simulink model "eVTOL_System"  (R2024b)
settings: Solver=FixedStepAuto  StartTime=0.0  StopTime=inf  RelTol=1e-3
undefined symbols (not defined in the file): airspeed, Battery, BCE12, BCE_Set_init, BMS_Controller_State, C, Cell10_P, Cell11_P, Cell12_P, Cell13_P, Cell14_P, Cell15_P, Cell16_P, Cell17_P, Cell18_P, Cell19_P, Cell1_N, Cell1_P, Cell20_P, Cell21_P, Cell22_P, Cell23_P, Cell24_P, Cell2_P, Cell3_P, Cell4_P, Cell5_P, Cell6_P, Cell7_P, Cell8_P, Cell9_P, Charging_State, CityMission, control, controlParams, ControlSampleTime, CriticalTiltAngle, currentFactor, CV_Gain, ddx, ddy, ddz, Device_01, Device_02, DiscIntNeverNeededParam, dx, dy, dz, Earth, env, F, F28379D_ADC_MaxCount, F28379D_ADC_Vmax, FixedWingMission, flightState, Foc_Ki_IxTcpu, Foc_Ki_S, Foc_Kp_I, Foc_Kp_S, fractalcoef ... (+68)
libraries: fl_lib x1115, nesl_utility x617, slrealtimeethercatlib x217, simulink x130, canmsglib x101, speedgoatlib_IO611_obsolete x91, slpidlib x49, mcbcontrolslib x44, slrealtimeutilitieslib x35, speedgoatlib_hdlCoder_IO3xx x31, dspstat3 x24, mcbpositiondecoderlib x12
(part 11 of 31)

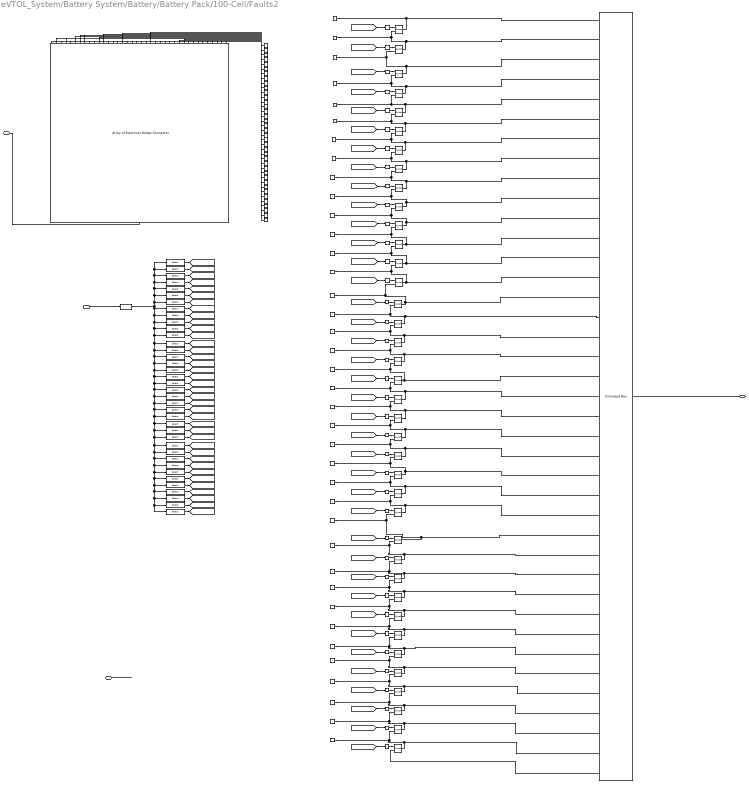
== system eVTOL_System/Battery System/Battery/Battery Pack/100-Cell/Faults2 ==
  note: Short-Circuits
  note: Short-Circuits
  note: Short-Circuits
  Short_Circuits : Inport
  Array of Electrical Nodes Connector2 : batt_lib/Connectors/Array of Electrical Nodes Connector  numInputConnections=simscape.battery.enum.thermal.numArrayOfNodesConnections.thirtyeight  inNode1NumElements=1  inNode2NumElements=1  inNode3NumElements=1  inNode4NumElements=1  inNode5NumElements=1  inNode6NumElements=1  inNode7NumElements=1  inNode8NumElements=1  inNode9NumElements=1  inNode10NumElements=1  inNode11NumElements=1  inNode12NumElements=1  inNode13NumElements=1  inNode14NumElements=1  inNode15NumElements=1  inNode16NumElements=1  inNode17NumElements=1  inNode18NumElements=1  inNode19NumElements=1  inNode20NumElements=1  inNode21NumElements=1  inNode22NumElements=1  inNode23NumElements=1  inNode24NumElements=1  inNode25NumElements=1  inNode26NumElements=1  inNode27NumElements=1  inNode28NumElements=1  inNode29NumElements=1  inNode30NumElements=1  inNode31NumElements=1  inNode32NumElements=1  inNode33NumElements=1  inNode34NumElements=1  inNode35NumElements=1  inNode36NumElements=1  inNode37NumElements=1  inNode38NumElements=1  inNode39NumElements=1  inNode40NumElements=1  inNode41NumElements=1  inNode42NumElements=1  inNode43NumElements=1  inNode44NumElements=1  inNode45NumElements=1  inNode46NumElements=1  inNode47NumElements=1  inNode48NumElements=1  inNode49NumElements=1  inNode50NumElements=1
      settings: InternalSimscapePortConfiguration="{\"Bottom\":[{\"id\":\"outConn\",\"label\":\"outConn\",\"type\":\"foundation.electrical.electrical\"}],\"Left\":[],\"Right\":[],\"Top\":[{\"id\":\"inConn1\",\"label\":\"inConn1\",\"type\":\"foundation.electrical.electrical\"},{\"id\":\"inConn2\",\"label\":\"inConn2\",\"type\":\"foundation.electrical.electrical\"},{\"id\":\"inConn3\",\"label\":\"inConn3\",\"type\":\"foundation.electrical.electrical\"},{\"id\":\"inConn4\",\"label\":\"inConn4\",\"type\":\"foundation.electrical.electrical\"},{\"id\":\"inConn5\",\"label\":\"inConn5\",\"type\":\"foundation.electrical.electrical\"},{\"id\":\"inConn6\",\"label\":\"inConn6\",\"type\":\"foundation.electrical.electrical\"},{\"id\":\"inConn7\",\"label\":\"inConn7\",\"type\":\"foundation.electrical.electrical\"},{\"id\":\"inConn8\",\"label\":\"inConn8\",\"type\":\"foundation.electrical.electrical\"},{\"id\":\"inConn9\",\"label\":\"inConn9\",\"type\":\"foundation.electrical.electrical\"},{\"id\":\"inConn10\",\"label\":\"inConn10\",\"type\":\"foundation.electrical.electrical\"},{\"id\":\"inConn11\",\"label\":\"inConn11\",\"type\":\"foundation.electrical.electrical\"},{\"id\":\"inConn12\",\"label\":\"inConn12\",\"type\":\"foundation.electrical.electrical\"},{\"id\":\"inConn13\",\"label\":\"inConn13\",\"type\":\"foundation.electrical.electrical\"},{\"id\":\"inConn14\",\"label\":\"inConn14\",\"type\":\"foundation.electrical.electrical\"},{\"id\":\"inConn15\",\"label\":\"inConn15\",\"type\":\"foundation.electrical.electrical\"},{\"id\":\"inConn16\",\"label\":\"inConn16\",\"type\":\"foundation.electrical.electrical\"},{\"id\":\"inConn17\",\"label\":\"inConn17\",\"type\":\"foundation.electrical.electrical\"},{\"id\":\"inConn18\",\"label\":\"inConn18\",\"type\":\"foundation.electrical.electrical\"},{\"id\":\"inConn19\",\"label\":\"inConn19\",\"type\":\"foundation.electrical.electrical\"},{\"id\":\"inConn20\",\"label\":\"inConn20\",\"type\":\"foundation.electrical.electrical\"},{\"id\":\"inConn21\",\"label\":\"inConn21\",\"type\":\"foundation.electrical.electrical\"},{\"id\":\"inConn22\",\"label\":\"inConn22\",\"type\":\"foundation.electrical.electrical\"},{\"id\":\"inConn23\",\"label\":\"inConn23\",\"type\":\"foundation.electrical.electrical\"},{\"id\":\"inConn24\",\"label\":\"inConn24\",\"type\":\"foundation.electrical.electrical\"},{\"id\":\"inConn25\",\"label\":\"inConn25\",\"type\":\"foundation.electrical.electrical\"},{\"id\":\"inConn26\",\"label\":\"inConn26\",\"type\":\"foundation.electrical.electrical\"},{\"id\":\"inConn27\",\"label\":\"inConn27\",\"type\":\"foundation.electrical.electrical\"},{\"id\":\"inConn28\",\"label\":\"inConn28\",\"type\":\"foundation.electrical.electrical\"},{\"id\":\"inConn29\",\"label\":\"inConn29\",\"type\":\"foundation.electrical.electrical\"},{\"id\":\"inConn30\",\"label\":\"inConn30\",\"type\":\"foundation.electrical.electrical\"},{\"id\":\"inConn31\",\"label\":\"inConn31\",\"type\":\"foundation.electrical.electrical\"},{\"id\":\"inConn32\",\"label\":\"inConn32\",\"type\":\"foundation.electrical.electrical\"},{\"id\":\"inConn33\",\"label\":\"inConn33\",\"type\":\"foundation.electrical.electrical\"},{\"id\":\"inConn34\",\"label\":\"inConn34\",\"type\":\"foundation.electrical.electrical\"},{\"id\":\"inConn35\",\"label\":\"inConn35\",\"type\":\"foundation.electrical.electrical\"},{\"id\":\"inConn36\",\"label\":\"inConn36\",\"type\":\"foundation.electrical.electrical\"},{\"id\":\"inConn37\",\"label\":\"inConn37\",\"type\":\"foundation.electrical.electrical\"},{\"id\":\"inConn38\",\"label\":\"inConn38\",\"type\":\"foundation.electrical.electrical\"}]}"
  Connection Label1 : ConnectionLabel  Label=pos12
  Connection Label10 : ConnectionLabel  Label=pos3
  Connection Label100 : ConnectionLabel  Label=pos1
  Connection Label101 : ConnectionLabel  Label=pos7
  Connection Label102 : ConnectionLabel  Label=pos3
  Connection Label103 : ConnectionLabel  Label=pos2
  Connection Label104 : ConnectionLabel  Label=pos8
  Connection Label105 : ConnectionLabel  Label=pos9
  Connection Label106 : ConnectionLabel  Label=pos10
  Connection Label107 : ConnectionLabel  Label=pos11
  Connection Label108 : ConnectionLabel  Label=pos12
  Connection Label109 : ConnectionLabel  Label=pos6
  Connection Label11 : ConnectionLabel  Label=pos2
  Connection Label110 : ConnectionLabel  Label=pos13
  Connection Label111 : ConnectionLabel  Label=pos19
  Connection Label112 : ConnectionLabel  Label=pos15
  Connection Label113 : ConnectionLabel  Label=pos14
  Connection Label114 : ConnectionLabel  Label=pos20
  Connection Label115 : ConnectionLabel  Label=pos21
  Connection Label116 : ConnectionLabel  Label=pos5
  Connection Label117 : ConnectionLabel  Label=pos22
  Connection Label118 : ConnectionLabel  Label=pos23
  Connection Label119 : ConnectionLabel  Label=pos24
  Connection Label12 : ConnectionLabel  Label=pos1
  Connection Label120 : ConnectionLabel  Label=pos18
  Connection Label121 : ConnectionLabel  Label=pos17
  Connection Label122 : ConnectionLabel  Label=pos16
  Connection Label123 : ConnectionLabel  Label=pos25
  Connection Label124 : ConnectionLabel  Label=pos31
  Connection Label125 : ConnectionLabel  Label=pos27
  Connection Label126 : ConnectionLabel  Label=pos26
  Connection Label127 : ConnectionLabel  Label=pos4
  Connection Label128 : ConnectionLabel  Label=pos32
  Connection Label129 : ConnectionLabel  Label=pos33
  Connection Label13 : ConnectionLabel  Label=pos24
  Connection Label130 : ConnectionLabel  Label=pos34
  Connection Label131 : ConnectionLabel  Label=pos35
  Connection Label132 : ConnectionLabel  Label=pos36
  Connection Label133 : ConnectionLabel  Label=pos30
  Connection Label134 : ConnectionLabel  Label=pos29
  Connection Label135 : ConnectionLabel  Label=pos28
  Connection Label136 : ConnectionLabel  Label=pos37
  Connection Label137 : ConnectionLabel  Label=pos38
  Connection Label14 : ConnectionLabel  Label=pos23
  Connection Label15 : ConnectionLabel  Label=pos22
  Connection Label16 : ConnectionLabel  Label=pos21
  Connection Label17 : ConnectionLabel  Label=pos20
  Connection Label18 : ConnectionLabel  Label=pos19
  Connection Label19 : ConnectionLabel  Label=pos18
  Connection Label2 : ConnectionLabel  Label=pos11
  Connection Label20 : ConnectionLabel  Label=pos17
  Connection Label21 : ConnectionLabel  Label=pos29
  Connection Label22 : ConnectionLabel  Label=pos16
  Connection Label23 : ConnectionLabel  Label=pos15
  Connection Label3 : ConnectionLabel  Label=pos10
  Connection Label4 : ConnectionLabel  Label=pos9
  Connection Label48 : ConnectionLabel  Label=pos14
  Connection Label49 : ConnectionLabel  Label=pos13
  Connection Label5 : ConnectionLabel  Label=pos8
  Connection Label50 : ConnectionLabel  Label=pos28
  Connection Label51 : ConnectionLabel  Label=pos27
  Connection Label52 : ConnectionLabel  Label=pos26
  Connection Label53 : ConnectionLabel  Label=pos25
  Connection Label54 : ConnectionLabel  Label=pos34
  Connection Label55 : ConnectionLabel  Label=pos33
  Connection Label56 : ConnectionLabel  Label=pos32
  Connection Label57 : ConnectionLabel  Label=pos31
  Connection Label58 : ConnectionLabel  Label=pos30
  Connection Label59 : ConnectionLabel  Label=pos38
  Connection Label6 : ConnectionLabel  Label=pos7
  Connection Label60 : ConnectionLabel  Label=pos37
  Connection Label61 : ConnectionLabel  Label=pos36
  Connection Label62 : ConnectionLabel  Label=pos35
  Connection Label7 : ConnectionLabel  Label=pos6
  Connection Label8 : ConnectionLabel  Label=pos5
  Connection Label9 : ConnectionLabel  Label=pos4
  Data Type Conversion2 : DataTypeConversion  OutDataTypeStr=double  SaturateOnIntegerOverflow=off  RndMeth=Floor
  Selector1 : Selector  IndexOptions=Index vector (dialog)  Indices=73  OutputSizes=1
  Selector10 : Selector  IndexOptions=Index vector (dialog)  Indices=63  OutputSizes=1
  Selector11 : Selector  IndexOptions=Index vector (dialog)  Indices=64  OutputSizes=1
  Selector12 : Selector  IndexOptions=Index vector (dialog)  Indices=66  OutputSizes=1
  Selector13 : Selector  IndexOptions=Index vector (dialog)  Indices=76  OutputSizes=1
  Selector14 : Selector  IndexOptions=Index vector (dialog)  Indices=86  OutputSizes=1
  Selector15 : Selector  IndexOptions=Index vector (dialog)  Indices=85  OutputSizes=1
  Selector16 : Selector  IndexOptions=Index vector (dialog)  Indices=83  OutputSizes=1
  Selector17 : Selector  IndexOptions=Index vector (dialog)  Indices=78  OutputSizes=1
  Selector18 : Selector  IndexOptions=Index vector (dialog)  Indices=77  OutputSizes=1
  Selector19 : Selector  IndexOptions=Index vector (dialog)  Indices=80  OutputSizes=1
  Selector2 : Selector  IndexOptions=Index vector (dialog)  Indices=71  OutputSizes=1
  Selector20 : Selector  IndexOptions=Index vector (dialog)  Indices=82  OutputSizes=1
  Selector21 : Selector  IndexOptions=Index vector (dialog)  Indices=75  OutputSizes=1
  Selector22 : Selector  IndexOptions=Index vector (dialog)  Indices=81  OutputSizes=1
  Selector23 : Selector  IndexOptions=Index vector (dialog)  Indices=79  OutputSizes=1
  Selector24 : Selector  IndexOptions=Index vector (dialog)  Indices=84  OutputSizes=1
  Selector25 : Selector  IndexOptions=Index vector (dialog)  Indices=89  OutputSizes=1
  Selector26 : Selector  IndexOptions=Index vector (dialog)  Indices=88  OutputSizes=1
  Selector27 : Selector  IndexOptions=Index vector (dialog)  Indices=91  OutputSizes=1
  Selector29 : Selector  IndexOptions=Index vector (dialog)  Indices=100  OutputSizes=1
  Selector3 : Selector  IndexOptions=Index vector (dialog)  Indices=72  OutputSizes=1
  Selector30 : Selector  IndexOptions=Index vector (dialog)  Indices=98  OutputSizes=1
  Selector31 : Selector  IndexOptions=Index vector (dialog)  Indices=93  OutputSizes=1
  Selector32 : Selector  IndexOptions=Index vector (dialog)  Indices=92  OutputSizes=1
  Selector33 : Selector  IndexOptions=Index vector (dialog)  Indices=95  OutputSizes=1
  Selector34 : Selector  IndexOptions=Index vector (dialog)  Indices=97  OutputSizes=1
  Selector35 : Selector  IndexOptions=Index vector (dialog)  Indices=90  OutputSizes=1
  Selector36 : Selector  IndexOptions=Index vector (dialog)  Indices=96  OutputSizes=1
  Selector37 : Selector  IndexOptions=Index vector (dialog)  Indices=94  OutputSizes=1
  Selector38 : Selector  IndexOptions=Index vector (dialog)  Indices=99  OutputSizes=1
  Selector39 : Selector  IndexOptions=Index vector (dialog)  Indices=87  OutputSizes=1
  Selector4 : Selector  IndexOptions=Index vector (dialog)  Indices=69  OutputSizes=1
  Selector5 : Selector  IndexOptions=Index vector (dialog)  Indices=67  OutputSizes=1
  Selector6 : Selector  IndexOptions=Index vector (dialog)  Indices=74  OutputSizes=1
  Selector7 : Selector  IndexOptions=Index vector (dialog)  Indices=68  OutputSizes=1
  Selector8 : Selector  IndexOptions=Index vector (dialog)  Indices=70  OutputSizes=1
  Selector9 : Selector  IndexOptions=Index vector (dialog)  Indices=65  OutputSizes=1
  Simscape Bus : SimscapeBus  HierarchyStrings=Cell38_P;Cell37_P;Cell36_P;Cell35_P;Cell34_P;Cell33_P;Cell32_P;Cell31_P;Cell30_P;Cell29_P;Cell28_P;Cell27_P;Cell26_P;Cell25_P;Cell24_P;Cell23_P;Cell22_P;Cell21_P;Cell20_P;Cell19_P;Cell18_P;Cell17_P;Cell16_P;Cell15_P;Cell14_P;Cell13_P;Cell12_P;Cell11_P;Cell10_P;Cell9_P;Cell8_P;Cell7_P;Cell6_P;Cell5_P;Cell4_P;Cell3_P;Cell2_P;Cell1_P;Cell1_N
  Simulink-PS Converter{1..38} (38 alike) : nesl_utility/Simulink-PS Converter  PhysicalDomain=network_engine_domain  SubClassName=ps_input  LeftPortType=input  RightPortType=output  PseudoPeriodic=off  Frequencies=[]  NoiseDistribution=none  NoiseParameters=[]  Unit=1  AffineConversion=off  FilteringAndDerivatives=zero  SimscapeFilterOrder=1  InputFilterTimeConstant=0.001  UdotUserProvided=1
  Switch{,1..37} (38 alike) : fl_lib/Electrical/Electrical Elements/Switch  R_closed=0.01 Ohm  G_open=1e-8 1/Ohm  Threshold=0.5  i_specify=off  i_priority=None  i=0 A  i_nominal_specify=off  i_nominal_value=1  i_nominal_unit=A  v_specify=off  v_priority=None  v=0 V  v_nominal_specify=off  v_nominal_value=1  v_nominal_unit=V
  +Bus : PMIOPort  Side=Right
  Cells : PMIOPort  Port=2  Side=Right
  =Bus : PMIOPort  Port=3  Side=Right
  wires:
  [Cell37_Switch_SC] -> Simulink-PS Converter24/1
  [Cell36_Switch_SC] -> Simulink-PS Converter23/1
  [Cell38_Switch_SC] -> Simulink-PS Converter25/1
  [Cell27_Switch_SC] -> Simulink-PS Converter14/1
  [Cell28_Switch_SC] -> Simulink-PS Converter15/1
  [Cell35_Switch_SC] -> Simulink-PS Converter22/1
  [Cell31_Switch_SC] -> Simulink-PS Converter18/1
  [Cell34_Switch_SC] -> Simulink-PS Converter21/1
  [Cell29_Switch_SC] -> Simulink-PS Converter16/1
  [Cell30_Switch_SC] -> Simulink-PS Converter17/1
  [Cell33_Switch_SC] -> Simulink-PS Converter20/1
  [Cell32_Switch_SC] -> Simulink-PS Converter19/1
  [Cell23_Switch_SC] -> Simulink-PS Converter9/1
  [Cell20_Switch_SC] -> Simulink-PS Converter6/1
  [Cell17_Switch_SC] -> Simulink-PS Converter3/1
  [Cell18_Switch_SC] -> Simulink-PS Converter4/1
  [Cell26_Switch_SC] -> Simulink-PS Converter12/1
  [Cell19_Switch_SC] -> Simulink-PS Converter5/1
  [Cell25_Switch_SC] -> Simulink-PS Converter11/1
  [Cell22_Switch_SC] -> Simulink-PS Converter8/1
  [Cell15_Switch_SC] -> Simulink-PS Converter1/1
  [Cell24_Switch_SC] -> Simulink-PS Converter10/1
  [Cell21_Switch_SC] -> Simulink-PS Converter7/1
  [Cell16_Switch_SC] -> Simulink-PS Converter2/1
  [Cell5_Switch_SC] -> Simulink-PS Converter30/1
  [Cell4_Switch_SC] -> Simulink-PS Converter29/1
  [Cell10_Switch_SC] -> Simulink-PS Converter35/1
  [Cell12_Switch_SC] -> Simulink-PS Converter26/1
  [Cell3_Switch_SC] -> Simulink-PS Converter13/1
  [Cell9_Switch_SC] -> Simulink-PS Converter34/1
  [Cell14_Switch_SC] -> Simulink-PS Converter28/1
  [Cell13_Switch_SC] -> Simulink-PS Converter27/1
  [Cell6_Switch_SC] -> Simulink-PS Converter31/1
  [Cell11_Switch_SC] -> Simulink-PS Converter36/1
  [Cell7_Switch_SC] -> Simulink-PS Converter32/1
  [Cell8_Switch_SC] -> Simulink-PS Converter33/1
  [Cell1_Switch_SC] -> Simulink-PS Converter37/1
  Short_Circuits/1 -> Data Type Conversion2/1
  Selector11/1 -> [Cell2_Switch_SC]
  Selector16/1 -> [Cell21_Switch_SC]
  Selector9/1 -> [Cell3_Switch_SC]
  Selector14/1 -> [Cell24_Switch_SC]
  Selector27/1 -> [Cell29_Switch_SC]
  Selector10/1 -> [Cell1_Switch_SC]
  Selector7/1 -> [Cell6_Switch_SC]
  Selector2/1 -> [Cell9_Switch_SC]
  Selector21/1 -> [Cell13_Switch_SC]
  Selector13/1 -> [Cell14_Switch_SC]
  Selector34/1 -> [Cell35_Switch_SC]
  Selector22/1 -> [Cell19_Switch_SC]
  Selector26/1 -> [Cell26_Switch_SC]
  Selector31/1 -> [Cell31_Switch_SC]
  Data Type Conversion2/1 -> Selector5/1, Selector12/1, Selector9/1, Selector11/1, Selector30/1, Selector29/1, Selector38/1, Selector34/1, Selector36/1, Selector33/1, Selector37/1, Selector31/1, Selector32/1, Selector27/1, Selector35/1, Selector25/1, Selector26/1, Selector39/1, Selector14/1, Selector15/1, Selector24/1, Selector16/1, Selector20/1, Selector22/1, Selector19/1, Selector23/1, Selector17/1, Selector18/1, Selector13/1, Selector21/1, Selector10/1, Selector4/1, Selector8/1, Selector2/1, Selector3/1, Selector1/1, Selector6/1, Selector7/1
  Selector35/1 -> [Cell28_Switch_SC]
  Selector25/1 -> [Cell27_Switch_SC]
  Selector36/1 -> [Cell34_Switch_SC]
  Selector18/1 -> [Cell15_Switch_SC]
  Selector33/1 -> [Cell33_Switch_SC]
  Selector39/1 -> [Cell25_Switch_SC]
  Selector17/1 -> [Cell16_Switch_SC]
  Selector37/1 -> [Cell32_Switch_SC]
  Selector32/1 -> [Cell30_Switch_SC]
  Selector24/1 -> [Cell22_Switch_SC]
  Selector30/1 -> [Cell36_Switch_SC]
  Selector38/1 -> [Cell37_Switch_SC]
  Selector23/1 -> [Cell17_Switch_SC]
  Selector20/1 -> [Cell20_Switch_SC]
  Selector19/1 -> [Cell18_Switch_SC]
  Selector29/1 -> [Cell38_Switch_SC]
  Selector15/1 -> [Cell23_Switch_SC]
  Selector6/1 -> [Cell12_Switch_SC]
  Selector5/1 -> [Cell5_Switch_SC]
  Selector12/1 -> [Cell4_Switch_SC]
  Selector8/1 -> [Cell8_Switch_SC]
  Selector4/1 -> [Cell7_Switch_SC]
  Selector1/1 -> [Cell11_Switch_SC]
  Selector3/1 -> [Cell10_Switch_SC]
  [Cell2_Switch_SC] -> Simulink-PS Converter38/1
  connections:
  Simulink-PS Converter17/RConn1 -- Switch3/RConn1
  Switch3/LConn1 -- Simscape Bus/LConn30 -- Switch2/RConn2 -- Connection Label58/LConn1
  Switch6/LConn1 -- Simscape Bus/LConn33 -- Switch5/RConn2 -- Connection Label55/LConn1
  Switch7/LConn1 -- Simscape Bus/LConn34 -- Connection Label54/LConn1 -- Switch6/RConn2
  Switch2/LConn1 -- Simscape Bus/LConn29 -- Switch1/RConn2 -- Connection Label21/LConn1
  Simulink-PS Converter16/RConn1 -- Switch2/RConn1
  Simulink-PS Converter19/RConn1 -- Switch5/RConn1
  Switch10/LConn1 -- Simscape Bus/LConn37 -- Switch9/RConn2 -- Connection Label60/LConn1
  Simulink-PS Converter25/RConn1 -- Switch11/RConn1
  Switch11/LConn1 -- Simscape Bus/LConn38 -- Connection Label59/LConn1 -- Switch10/RConn2
  Switch9/LConn1 -- Simscape Bus/LConn36 -- Switch8/RConn2 -- Connection Label61/LConn1
  Simulink-PS Converter14/RConn1 -- Switch/RConn1
  Simscape Bus/LConn39 -- Switch11/RConn2
  Simulink-PS Converter18/RConn1 -- Switch4/RConn1
  Switch4/LConn1 -- Simscape Bus/LConn31 -- Switch3/RConn2 -- Connection Label57/LConn1
  Simulink-PS Converter24/RConn1 -- Switch10/RConn1
  Switch8/LConn1 -- Simscape Bus/LConn35 -- Switch7/RConn2 -- Connection Label62/LConn1
  Simulink-PS Converter20/RConn1 -- Switch6/RConn1
  Simulink-PS Converter15/RConn1 -- Switch1/RConn1
  Simulink-PS Converter21/RConn1 -- Switch7/RConn1
  Simulink-PS Converter23/RConn1 -- Switch9/RConn1
  Simulink-PS Converter22/RConn1 -- Switch8/RConn1
  Switch5/LConn1 -- Simscape Bus/LConn32 -- Switch4/RConn2 -- Connection Label56/LConn1
  Simscape Bus/LConn27 -- Connection Label51/LConn1 -- Switch15/RConn2 -- Switch/LConn1
  Switch1/LConn1 -- Simscape Bus/LConn28 -- Connection Label50/LConn1 -- Switch/RConn2
  =Bus/RConn1 -- ?
  Switch17/LConn1 -- Simscape Bus/LConn18 -- Switch16/RConn2 -- Connection Label19/LConn1
  Switch14/LConn1 -- Simscape Bus/LConn25 -- Switch23/RConn2 -- Connection Label53/LConn1
  Switch19/LConn1 -- Connection Label17/LConn1 -- Switch18/RConn2 -- Simscape Bus/LConn20
  Switch13/LConn1 -- Simscape Bus/LConn16 -- Switch12/RConn2 -- Connection Label22/LConn1
  Switch22/LConn1 -- Simscape Bus/LConn23 -- Connection Label14/LConn1 -- Switch21/RConn2
  Switch18/LConn1 -- Simscape Bus/LConn19 -- Connection Label18/LConn1 -- Switch17/RConn2
  Switch16/LConn1 -- Simscape Bus/LConn17 -- Connection Label20/LConn1 -- Switch13/RConn2
  Switch12/LConn1 -- Switch27/RConn2 -- Connection Label23/LConn1 -- Simscape Bus/LConn15
  Switch21/LConn1 -- Switch20/RConn2 -- Connection Label15/LConn1 -- Simscape Bus/LConn22
  Simscape Bus/LConn21 -- Switch19/RConn2 -- Connection Label16/LConn1 -- Switch20/LConn1
  Simulink-PS Converter12/RConn1 -- Switch15/RConn1
  Simulink-PS Converter7/RConn1 -- Switch20/RConn1
  Simulink-PS Converter10/RConn1 -- Switch23/RConn1
  Simulink-PS Converter2/RConn1 -- Switch13/RConn1
  Simulink-PS Converter3/RConn1 -- Switch16/RConn1
  Simulink-PS Converter1/RConn1 -- Switch12/RConn1
  Simulink-PS Converter11/RConn1 -- Switch14/RConn1
  Simulink-PS Converter8/RConn1 -- Switch21/RConn1
  Simulink-PS Converter9/RConn1 -- Switch22/RConn1
  Simulink-PS Converter5/RConn1 -- Switch18/RConn1
  Simulink-PS Converter6/RConn1 -- Switch19/RConn1
  Simulink-PS Converter4/RConn1 -- Switch17/RConn1
  Switch15/LConn1 -- Simscape Bus/LConn26 -- Connection Label52/LConn1 -- Switch14/RConn2
  Simscape Bus/LConn24 -- Switch23/LConn1 -- Connection Label13/LConn1 -- Switch22/RConn2
  Cells/RConn1 -- Simscape Bus/RConn1
  Switch33/LConn1 -- Connection Label3/LConn1 -- Switch32/RConn2 -- Simscape Bus/LConn10
  Simscape Bus/LConn3 -- Connection Label10/LConn1 -- Switch37/RConn2 -- Switch24/LConn1
  Switch34/LConn1 -- Simscape Bus/LConn11 -- Connection Label2/LConn1 -- Switch33/RConn2
  Switch25/LConn1 -- Connection Label9/LConn1 -- Switch24/RConn2 -- Simscape Bus/LConn4
  Switch31/LConn1 -- Switch30/RConn2 -- Connection Label5/LConn1 -- Simscape Bus/LConn8
  Simscape Bus/LConn14 -- Switch27/LConn1 -- Switch26/RConn2 -- Connection Label48/LConn1
  Switch26/LConn1 -- Connection Label49/LConn1 -- Switch35/RConn2 -- Simscape Bus/LConn13
  Switch30/LConn1 -- Switch29/RConn2 -- Connection Label6/LConn1 -- Simscape Bus/LConn7
  Switch32/LConn1 -- Switch31/RConn2 -- Connection Label4/LConn1 -- Simscape Bus/LConn9
  Switch29/LConn1 -- Connection Label7/LConn1 -- Switch28/RConn2 -- Simscape Bus/LConn6
  Switch28/LConn1 -- Switch25/RConn2 -- Connection Label8/LConn1 -- Simscape Bus/LConn5
  Switch35/LConn1 -- Connection Label1/LConn1 -- Switch34/RConn2 -- Simscape Bus/LConn12
  Simulink-PS Converter31/RConn1 -- Switch29/RConn1
  Simulink-PS Converter13/RConn1 -- Switch24/RConn1
  Simulink-PS Converter28/RConn1 -- Switch27/RConn1
  Simulink-PS Converter35/RConn1 -- Switch33/RConn1
  Simulink-PS Converter34/RConn1 -- Switch32/RConn1
  Simulink-PS Converter33/RConn1 -- Switch31/RConn1
  Simulink-PS Converter27/RConn1 -- Switch26/RConn1
  Simulink-PS Converter32/RConn1 -- Switch30/RConn1
  Simulink-PS Converter29/RConn1 -- Switch25/RConn1
  Simulink-PS Converter36/RConn1 -- Switch34/RConn1
  Simulink-PS Converter30/RConn1 -- Switch28/RConn1
  Simulink-PS Converter26/RConn1 -- Switch35/RConn1
  Simscape Bus/LConn1 -- Connection Label12/LConn1 -- Switch36/LConn1
  Switch37/LConn1 -- Connection Label11/LConn1 -- Switch36/RConn2 -- Simscape Bus/LConn2
  Simulink-PS Converter37/RConn1 -- Switch36/RConn1
  Simulink-PS Converter38/RConn1 -- Switch37/RConn1
  Connection Label132/LConn1 -- Array of Electrical Nodes Connector2/LConn36
  Connection Label107/LConn1 -- Array of Electrical Nodes Connector2/LConn11
  Connection Label106/LConn1 -- Array of Electrical Nodes Connector2/LConn10
  Connection Label136/LConn1 -- Array of Electrical Nodes Connector2/LConn37
  Connection Label131/LConn1 -- Array of Electrical Nodes Connector2/LConn35
  Connection Label135/LConn1 -- Array of Electrical Nodes Connector2/LConn28
  Connection Label129/LConn1 -- Array of Electrical Nodes Connector2/LConn33
  Connection Label128/LConn1 -- Array of Electrical Nodes Connector2/LConn32
  Connection Label124/LConn1 -- Array of Electrical Nodes Connector2/LConn31
  Connection Label125/LConn1 -- Array of Electrical Nodes Connector2/LConn27
  Connection Label118/LConn1 -- Array of Electrical Nodes Connector2/LConn23
  Connection Label121/LConn1 -- Array of Electrical Nodes Connector2/LConn17
  Connection Label114/LConn1 -- Array of Electrical Nodes Connector2/LConn20
  Connection Label102/LConn1 -- Array of Electrical Nodes Connector2/LConn3
  Connection Label133/LConn1 -- Array of Electrical Nodes Connector2/LConn30
  Connection Label120/LConn1 -- Array of Electrical Nodes Connector2/LConn18
  Connection Label123/LConn1 -- Array of Electrical Nodes Connector2/LConn25
  Connection Label115/LConn1 -- Array of Electrical Nodes Connector2/LConn21
  Connection Label111/LConn1 -- Array of Electrical Nodes Connector2/LConn19
  Connection Label112/LConn1 -- Array of Electrical Nodes Connector2/LConn15
  Connection Label126/LConn1 -- Array of Electrical Nodes Connector2/LConn26
  Connection Label104/LConn1 -- Array of Electrical Nodes Connector2/LConn8
  Connection Label109/LConn1 -- Array of Electrical Nodes Connector2/LConn6
  Connection Label119/LConn1 -- Array of Electrical Nodes Connector2/LConn24
  Connection Label105/LConn1 -- Array of Electrical Nodes Connector2/LConn9
  Connection Label116/LConn1 -- Array of Electrical Nodes Connector2/LConn5
  Connection Label137/LConn1 -- Array of Electrical Nodes Connector2/LConn38
  Connection Label100/LConn1 -- Array of Electrical Nodes Connector2/LConn1
  Connection Label134/LConn1 -- Array of Electrical Nodes Connector2/LConn29
  Connection Label122/LConn1 -- Array of Electrical Nodes Connector2/LConn16
  Connection Label103/LConn1 -- Array of Electrical Nodes Connector2/LConn2
  Connection Label117/LConn1 -- Array of Electrical Nodes Connector2/LConn22
  Connection Label101/LConn1 -- Array of Electrical Nodes Connector2/LConn7
  Connection Label127/LConn1 -- Array of Electrical Nodes Connector2/LConn4
  Connection Label130/LConn1 -- Array of Electrical Nodes Connector2/LConn34
  +Bus/RConn1 -- Array of Electrical Nodes Connector2/RConn1
  Connection Label113/LConn1 -- Array of Electrical Nodes Connector2/LConn14
  Connection Label110/LConn1 -- Array of Electrical Nodes Connector2/LConn13
  Connection Label108/LConn1 -- Array of Electrical Nodes Connector2/LConn12

== system eVTOL_System/Battery System/Battery/Battery Pack/100-Cell/Trigger_Faults ==
  Cell_Number : Constant  Value=12
  Delay : Delay  DelayLength=1
  Enable : Constant  Value=0
  Reset : Constant  Value=0
  Short-Circuit_Faults : MATLAB Function  TreatAsAtomicUnit=on
  ShortCircuit : Outport
  wires:
  Short-Circuit_Faults/1(ShortCircuit) -> Delay/1, ShortCircuit/1
  Cell_Number/1 -> Short-Circuit_Faults/1(CellNumber)
  Enable/1 -> Short-Circuit_Faults/2(Enable)
  Reset/1 -> Short-Circuit_Faults/3(Reset)
  Delay/1 -> Short-Circuit_Faults/4(Feedback)

== system eVTOL_System/Battery System/Battery/HW Interface/BCE - HIL/Battery Cell Emulator ==
  Sensor_Values_Sim : Inport
  "BCE Bus Packing " : Subsystem
  BCE Bus Packing 1 : Subsystem
  "BCE Read " : Subsystem  InitFcn=sg_bce.checkNumberOfBlocksGlobal(bdroot);  mask(bce_read){}
      settings: OpenFcn=sg_bce.openFcnRead;
      mask Help: eval('sg.utils.help.show(''io_main/refentry_bce_read'');')
      mask Display: disp('Speedgoat\nBMTS Read\nEtherCAT Bus: 0, Device: 1\nBCE12-0505');port_label('output',1,'Data');
  BCE Read 1 : Subsystem  InitFcn=sg_bce.checkNumberOfBlocksGlobal(bdroot);  mask(bce_read){}
      settings: OpenFcn=sg_bce.openFcnRead;
      mask Help: eval('sg.utils.help.show(''io_main/refentry_bce_read'');')
      mask Display: disp('Speedgoat\nBMTS Read\nEtherCAT Bus: 0, Device: 2\nBCE12-0505');port_label('output',1,'Data');
  "BCE Setup " : Subsystem  LoadFcn=|  InitFcn=|  mask(bce_setup){}
      LoadFcn=|
      | sg_bce.createBusSignals;
      | sg_bce.setupEniCallback(gcb, bdroot);
      InitFcn=|
      | sg_bce.createBusSignals;
      | sg_bce.checkNumberOfBlocksGlobal(bdroot);
      | sg_bce.setupEniCallback(gcb, bdroot);
      settings: OpenFcn=sg_bce.openFcnSetup;
      mask Help: eval('sg.utils.help.show(''io_main/refentry_bce_setup'');')
      mask Display: disp('Speedgoat\nBattery Management Testing Systems\nEtherCAT Bus: 0\nSetup');
  "BCE Write " : Subsystem  InitFcn=sg_bce.checkNumberOfBlocksGlobal(bdroot);  mask(bce_write){}
      settings: OpenFcn=sg_bce.openFcnWrite;
      mask Help: eval('sg.utils.help.show(''io_main/refentry_bce_write'');')
      mask Display: disp('Speedgoat\nBMTS Write\nEtherCAT Bus: 0, Device: 1\nBCE12-0505');port_label('input',1,'Data');
  BCE Write 1 : Subsystem  InitFcn=sg_bce.checkNumberOfBlocksGlobal(bdroot);  mask(bce_write){}
      settings: OpenFcn=sg_bce.openFcnWrite;
      mask Help: eval('sg.utils.help.show(''io_main/refentry_bce_write'');')
      mask Display: disp('Speedgoat\nBMTS Write\nEtherCAT Bus: 0, Device: 2\nBCE12-0505');port_label('input',1,'Data');
  BCE_Init : Switch  Criteria=u2 > Threshold  SaturateOnIntegerOverflow=off  InputSameDT=off
  Bus Selector : BusSelector  OutputSignals=Cell_12.I,Cell_11.I,Cell_10.I,Cell_9.I,Cell_8.I,Cell_7.I,Cell_6.I,Cell_5.I,Cell_4.I,Cell_3.I,Cell_2.I,Cell_1.I
  Bus Selector2 : BusSelector  OutputSignals=Cell_12.V,Cell_11.V,Cell_10.V,Cell_9.V,Cell_8.V,Cell_7.V,Cell_6.V,Cell_5.V,Cell_4.V,Cell_3.V,Cell_2.V,Cell_1.V
  Bus Selector3 : BusSelector  OutputSignals=Cell_12.I,Cell_11.I,Cell_10.I,Cell_9.I,Cell_8.I,Cell_7.I,Cell_6.I,Cell_5.I,Cell_4.I,Cell_3.I,Cell_2.I,Cell_1.I
  Bus Selector4 : BusSelector  OutputSignals=Cell_12.V,Cell_11.V,Cell_10.V,Cell_9.V,Cell_8.V,Cell_7.V,Cell_6.V,Cell_5.V,Cell_4.V,Cell_3.V,Cell_2.V,Cell_1.V
  Constant : Constant  Value=[0 0 0 0 0 0 0 0 0 0 0 0 0 0 0 0 0 0 0 0 0 0 0 0]
  Data Type Conversion : DataTypeConversion  OutDataTypeStr=single  SaturateOnIntegerOverflow=off  RndMeth=Floor
  Data Type Conversion1 : DataTypeConversion  OutDataTypeStr=boolean  SaturateOnIntegerOverflow=off  RndMeth=Floor
  Data Type Conversion2 : DataTypeConversion  OutDataTypeStr=single  SaturateOnIntegerOverflow=off  RndMeth=Floor
  Data Type Conversion3 : DataTypeConversion  OutDataTypeStr=single  SaturateOnIntegerOverflow=off  RndMeth=Floor
  Data Type Conversion4 : DataTypeConversion  OutDataTypeStr=boolean  SaturateOnIntegerOverflow=off  RndMeth=Floor
  Demux : Demux  Outputs=12
  Demux1 : Demux  Outputs=12
  Enable : Constant
  Enable1 : Constant
  Mux{,1..3} (4 alike) : Mux  Inputs=12
  Mux4 : Mux  Inputs=2
  Mux5 : Mux  Inputs=2
  No_current : Constant  Value=0
  No_current1 : Constant  Value=0
  Selector : Subsystem
  Selector1 : Subsystem
  Selector2 : Subsystem
  Selector3 : Subsystem
  Step : Step  Time=2
  Current_Values : Outport
  Cell_Voltages : Outport  Port=2
  OtherVoltages : Outport  Port=3
  wires:
  "BCE Read "/1(Data) -> Bus Selector/1, Bus Selector2/1
  Constant/1 -> Data Type Conversion2/1
  Step/1 -> BCE_Init/2
  "BCE Bus Packing "/1(BCE Bus) -> "BCE Write "/1(Data)
  No_current/1 -> Data Type Conversion/1
  Data Type Conversion2/1 -> BCE_Init/3
  Bus Selector/1 -> Mux/1  "<I>"
  Bus Selector/2 -> Mux/2  "<I>"
  Bus Selector/3 -> Mux/3  "<I>"
  Bus Selector/4 -> Mux/4  "<I>"
  Bus Selector/5 -> Mux/5  "<I>"
  Bus Selector/6 -> Mux/6  "<I>"
  Bus Selector/7 -> Mux/7  "<I>"
  Bus Selector/8 -> Mux/8  "<I>"
  Bus Selector/9 -> Mux/9  "<I>"
  Bus Selector/10 -> Mux/10  "<I>"
  Bus Selector/11 -> Mux/11  "<I>"
  Bus Selector/12 -> Mux/12  "<I>"
  Bus Selector2/1 -> Mux1/1  "<V>"
  Bus Selector2/2 -> Mux1/2  "<V>"
  Bus Selector2/3 -> Mux1/3  "<V>"
  Bus Selector2/4 -> Mux1/4  "<V>"
  Bus Selector2/5 -> Mux1/5  "<V>"
  Bus Selector2/6 -> Mux1/6  "<V>"
  Bus Selector2/7 -> Mux1/7  "<V>"
  Bus Selector2/8 -> Mux1/8  "<V>"
  Bus Selector2/9 -> Mux1/9  "<V>"
  Bus Selector2/10 -> Mux1/10  "<V>"
  Bus Selector2/11 -> Mux1/11  "<V>"
  Bus Selector2/12 -> Mux1/12  "<V>"
  Enable/1 -> Data Type Conversion1/1
  Data Type Conversion1/1 -> "BCE Bus Packing "/1(Cell 1 Enable), "BCE Bus Packing "/9(Cell 9 Enable), "BCE Bus Packing "/12(Cell 12 Enable), "BCE Bus Packing "/11(Cell 11 Enable), "BCE Bus Packing "/10(Cell 10 Enable), "BCE Bus Packing "/8(Cell 8 Enable), "BCE Bus Packing "/7(Cell 7 Enable), "BCE Bus Packing "/6(Cell 6 Enable), "BCE Bus Packing "/5(Cell 5 Enable), "BCE Bus Packing "/4(Cell 4 Enable), "BCE Bus Packing "/3(Cell 3 Enable), "BCE Bus Packing "/2(Cell 2 Enable)
  Data Type Conversion/1 -> "BCE Bus Packing "/29(Cell 5 Current), "BCE Bus Packing "/28(Cell 4 Current), "BCE Bus Packing "/25(Cell 1 Current), "BCE Bus Packing "/26(Cell 2 Current), "BCE Bus Packing "/27(Cell 3 Current), "BCE Bus Packing "/30(Cell 6 Current), "BCE Bus Packing "/31(Cell 7 Current), "BCE Bus Packing "/32(Cell 8 Current), "BCE Bus Packing "/33(Cell 9 Current), "BCE Bus Packing "/34(Cell 10 Current), "BCE Bus Packing "/35(Cell 11 Current), "BCE Bus Packing "/36(Cell 12 Current)
  Demux/1 -> "BCE Bus Packing "/13(Cell 12 Voltage)
  Demux/2 -> "BCE Bus Packing "/14(Cell 11 Voltage)
  Demux/3 -> "BCE Bus Packing "/15(Cell 10 Voltage)
  Demux/4 -> "BCE Bus Packing "/16(Cell 9 Voltage)
  Demux/5 -> "BCE Bus Packing "/17(Cell 8 Voltage)
  Demux/6 -> "BCE Bus Packing "/18(Cell 7 Voltage)
  Demux/7 -> "BCE Bus Packing "/19(Cell 6 Voltage)
  Demux/8 -> "BCE Bus Packing "/20(Cell 5 Voltage)
  Demux/9 -> "BCE Bus Packing "/21(Cell 4 Voltage)
  Demux/10 -> "BCE Bus Packing "/22(Cell 3 Voltage)
  Demux/11 -> "BCE Bus Packing "/23(Cell 2 Voltage)
  Demux/12 -> "BCE Bus Packing "/24(Cell 1 Voltage)
  Demux1/3 -> BCE Bus Packing 1/15(Cell 10 Voltage)
  Data Type Conversion4/1 -> BCE Bus Packing 1/1(Cell 1 Enable), BCE Bus Packing 1/9(Cell 9 Enable), BCE Bus Packing 1/12(Cell 12 Enable), BCE Bus Packing 1/11(Cell 11 Enable), BCE Bus Packing 1/10(Cell 10 Enable), BCE Bus Packing 1/8(Cell 8 Enable), BCE Bus Packing 1/7(Cell 7 Enable), BCE Bus Packing 1/6(Cell 6 Enable), BCE Bus Packing 1/5(Cell 5 Enable), BCE Bus Packing 1/4(Cell 4 Enable), BCE Bus Packing 1/3(Cell 3 Enable), BCE Bus Packing 1/2(Cell 2 Enable)
  Demux1/5 -> BCE Bus Packing 1/17(Cell 8 Voltage)
  Enable1/1 -> Data Type Conversion4/1
  BCE Bus Packing 1/1(BCE Bus) -> BCE Write 1/1(Data)
  Demux1/4 -> BCE Bus Packing 1/16(Cell 9 Voltage)
  Demux1/1 -> BCE Bus Packing 1/13(Cell 12 Voltage)
  Demux1/12 -> BCE Bus Packing 1/24(Cell 1 Voltage)
  Demux1/11 -> BCE Bus Packing 1/23(Cell 2 Voltage)
  Demux1/10 -> BCE Bus Packing 1/22(Cell 3 Voltage)
  Demux1/7 -> BCE Bus Packing 1/19(Cell 6 Voltage)
  Demux1/9 -> BCE Bus Packing 1/21(Cell 4 Voltage)
  Data Type Conversion3/1 -> BCE Bus Packing 1/29(Cell 5 Current), BCE Bus Packing 1/28(Cell 4 Current), BCE Bus Packing 1/25(Cell 1 Current), BCE Bus Packing 1/26(Cell 2 Current), BCE Bus Packing 1/27(Cell 3 Current), BCE Bus Packing 1/30(Cell 6 Current), BCE Bus Packing 1/31(Cell 7 Current), BCE Bus Packing 1/32(Cell 8 Current), BCE Bus Packing 1/33(Cell 9 Current), BCE Bus Packing 1/34(Cell 10 Current), BCE Bus Packing 1/35(Cell 11 Current), BCE Bus Packing 1/36(Cell 12 Current)
  Demux1/2 -> BCE Bus Packing 1/14(Cell 11 Voltage)
  Demux1/6 -> BCE Bus Packing 1/18(Cell 7 Voltage)
  Demux1/8 -> BCE Bus Packing 1/20(Cell 5 Voltage)
  No_current1/1 -> Data Type Conversion3/1
  BCE_Init/1 -> Selector1/1(In1), Selector/1(In1)
  Bus Selector4/1 -> Mux3/1  "<V>"
  Bus Selector3/9 -> Mux2/9  "<I>"
  Bus Selector3/12 -> Mux2/12  "<I>"
  Bus Selector4/5 -> Mux3/5  "<V>"
  Bus Selector3/11 -> Mux2/11  "<I>"
  Bus Selector4/6 -> Mux3/6  "<V>"
  Mux3/1 -> [V2]
  Bus Selector3/4 -> Mux2/4  "<I>"
  Bus Selector4/12 -> Mux3/12  "<V>"
  Bus Selector4/11 -> Mux3/11  "<V>"
  Bus Selector3/7 -> Mux2/7  "<I>"
  Bus Selector3/2 -> Mux2/2  "<I>"
  Bus Selector3/3 -> Mux2/3  "<I>"
  Bus Selector3/5 -> Mux2/5  "<I>"
  Bus Selector3/6 -> Mux2/6  "<I>"
  Bus Selector4/8 -> Mux3/8  "<V>"
  Bus Selector3/1 -> Mux2/1  "<I>"
  Bus Selector3/10 -> Mux2/10  "<I>"
  Bus Selector3/8 -> Mux2/8  "<I>"
  Bus Selector4/9 -> Mux3/9  "<V>"
  BCE Read 1/1(Data) -> Bus Selector3/1, Bus Selector4/1
  Bus Selector4/7 -> Mux3/7  "<V>"
  Bus Selector4/2 -> Mux3/2  "<V>"
  Mux2/1 -> [I2]
  Bus Selector4/4 -> Mux3/4  "<V>"
  Bus Selector4/10 -> Mux3/10  "<V>"
  Bus Selector4/3 -> Mux3/3  "<V>"
  Mux/1 -> [I1]
  Mux1/1 -> [V1]
  Mux4/1 -> Current_Values/1
  Mux5/1 -> Cell_Voltages/1
  [I2] -> Mux4/2
  [I1] -> Mux4/1
  [V1] -> Mux5/1
  [V2] -> Mux5/2
  Selector2/1(Out1) -> BCE_Init/1
  Selector/1(Out1) -> Demux/1
  Selector1/1(Out1) -> Demux1/1
  Sensor_Values_Sim/1 -> Selector3/1(In1), Selector2/1(In1)
  Selector3/1(Out1) -> OtherVoltages/1

== system eVTOL_System/Battery System/Battery/HW Interface/BCE - HIL/Selector1 ==
  24Cells : Inport
  76Cells : Inport  Port=2
  Demux : Demux  Outputs=24
  Demux1 : Demux  Outputs=76
  Mux : Mux  Inputs=100
  100Cells : Outport
  wires:
  Demux/1 -> Mux/1
  Demux/2 -> Mux/2
  Demux/3 -> Mux/3
  Demux/4 -> Mux/4
  Demux/5 -> Mux/5
  Demux/6 -> Mux/6
  Demux/7 -> Mux/7
  Demux/8 -> Mux/8
  Demux/9 -> Mux/9
  Demux/10 -> Mux/10
  Demux/11 -> Mux/11
  Demux/12 -> Mux/12
  Demux/13 -> Mux/13
  Demux/14 -> Mux/14
  Demux/15 -> Mux/15
  Demux/16 -> Mux/16
  Demux/17 -> Mux/17
  Demux/18 -> Mux/18
  Demux/19 -> Mux/19
  Demux/20 -> Mux/20
  Demux/21 -> Mux/21
  Demux/22 -> Mux/22
  Demux/23 -> Mux/23
  Demux/24 -> Mux/24
  Demux1/1 -> Mux/25
  Demux1/2 -> Mux/26
  Demux1/3 -> Mux/27
  Demux1/4 -> Mux/28
  Demux1/5 -> Mux/29
  Demux1/6 -> Mux/30
  Demux1/7 -> Mux/31
  Demux1/8 -> Mux/32
  Demux1/9 -> Mux/33
  Demux1/10 -> Mux/34
  Demux1/11 -> Mux/35
  Demux1/12 -> Mux/36
  Demux1/13 -> Mux/37
  Demux1/14 -> Mux/38
  Demux1/15 -> Mux/39
  Demux1/16 -> Mux/40
  Demux1/17 -> Mux/41
  Demux1/18 -> Mux/42
  Demux1/19 -> Mux/43
  Demux1/20 -> Mux/44
  Demux1/21 -> Mux/45
  Demux1/22 -> Mux/46
  Demux1/23 -> Mux/47
  Demux1/24 -> Mux/48
  Demux1/25 -> Mux/49
  Demux1/26 -> Mux/50
  Demux1/27 -> Mux/51
  Demux1/28 -> Mux/52
  Demux1/29 -> Mux/53
  Demux1/30 -> Mux/54
  Demux1/31 -> Mux/55
  Demux1/32 -> Mux/56
  Demux1/33 -> Mux/57
  Demux1/34 -> Mux/58
  Demux1/35 -> Mux/59
  Demux1/36 -> Mux/60
  Demux1/37 -> Mux/61
  Demux1/38 -> Mux/62
  Demux1/39 -> Mux/63
  Demux1/40 -> Mux/64
  Demux1/41 -> Mux/65
  Demux1/42 -> Mux/66
  Demux1/43 -> Mux/67
  Demux1/44 -> Mux/68
  Demux1/45 -> Mux/69
  Demux1/46 -> Mux/70
  Demux1/47 -> Mux/71
  Demux1/48 -> Mux/72
  Demux1/49 -> Mux/73
  Demux1/50 -> Mux/74
  Demux1/51 -> Mux/75
  Demux1/52 -> Mux/76
  Demux1/53 -> Mux/77
  Demux1/54 -> Mux/78
  Demux1/55 -> Mux/79
  Demux1/56 -> Mux/80
  Demux1/57 -> Mux/81
  Demux1/58 -> Mux/82
  Demux1/59 -> Mux/83
  Demux1/60 -> Mux/84
  Demux1/61 -> Mux/85
  Demux1/62 -> Mux/86
  Demux1/63 -> Mux/87
  Demux1/64 -> Mux/88
  Demux1/65 -> Mux/89
  Demux1/66 -> Mux/90
  Demux1/67 -> Mux/91
  Demux1/68 -> Mux/92
  Demux1/69 -> Mux/93
  Demux1/70 -> Mux/94
  Demux1/71 -> Mux/95
  Demux1/72 -> Mux/96
  Demux1/73 -> Mux/97
  Demux1/74 -> Mux/98
  Demux1/75 -> Mux/99
  Demux1/76 -> Mux/100
  24Cells/1 -> Demux/1
  76Cells/1 -> Demux1/1
  Mux/1 -> 100Cells/1

== system eVTOL_System/Battery System/Battery/HW Interface/BCE - HIL/Shunt Emulator ==
  note: Shunt Emulator Blocks
  Sensor_Values_Sim : Inport
  Bus Selector : BusSelector  OutputSignals=Pack_Current
  Pack_Current : Outport
  wires:
  Sensor_Values_Sim/1 -> Bus Selector/1
  Bus Selector/1 -> Pack_Current/1  "<Pack_Current>"

== system eVTOL_System/Battery System/Battery/HW Interface/BCE - HIL/Temperature Emulator ==
  note: Temperature Emulation Blocks
  Sensor_Values_Sim : Inport
  Bus Selector : BusSelector  OutputSignals=Cell_Temperatures
  Cell_Temperatures : Outport
  wires:
  Sensor_Values_Sim/1 -> Bus Selector/1
  Bus Selector/1 -> Cell_Temperatures/1  "<Cell_Temperatures>"

== system eVTOL_System/Battery System/Instrumentation/Instrumented Signals/100-Cell/Celsius_to_Kelvin ==
  K : Inport
  Add : Sum  Inputs=+-
  Constant4 : Constant  Value=273.15
  C : Outport
  wires:
  Constant4/1 -> Add/2
  K/1 -> Add/1
  Add/1 -> C/1

== system eVTOL_System/Dynamics/Force and Moments/Aerodynamic Forces/Compute Body Frame Forces and Moments/Rotate FM to body frame ==
  FM_w : Inport
  alpha_beta : Inport  Port=2
  Forces : Selector  InputPortWidth=6  IndexOptions=Index vector (dialog)  Indices=[1 2 3]  OutputSizes=[(-2)]
  Moments : Selector  InputPortWidth=6  IndexOptions=Index vector (dialog)  Indices=[4 5 6]  OutputSizes=[(-2)]
  Rotate Forces : Subsystem
  Rotate Moments : Subsystem
  F_b : Outport  VectorParamsAs1DForOutWhenUnconnected=off
  M_b : Outport  Port=2  VectorParamsAs1DForOutWhenUnconnected=off
  wires:
  alpha_beta/1 -> Rotate Forces/2(alpha_beta), Rotate Moments/1(alpha_beta)
  Moments/1 -> Rotate Moments/2(M_w)
  FM_w/1 -> Moments/1, Forces/1
  Forces/1 -> Rotate Forces/1(F_w)
  Rotate Moments/1(M_b) -> M_b/1
  Rotate Forces/1(F_b) -> F_b/1

== system eVTOL_System/Dynamics/Force and Moments/Aerodynamic Forces/Compute Body Frame Forces and Moments/Wind frame F& M ==
  Airdata : Inport
  CtrlSurfaces : Inport  Port=2
  p,q,r : Inport  Port=3
  Bus Creator1 : BusCreator  Inputs=2
  Bus Selector1 : BusSelector  OutputSignals=dA,dR
  Bus Selector2 : BusSelector  OutputSignals=dE,dA,dR
  Bus Selector6 : BusSelector  OutputSignals=beta,airspeed
  Bus Selector7 : BusSelector  OutputSignals=alpha,airspeed
  Get Forces and Moments : Subsystem
  Lateral Channel : Subsystem
  Longitudinal Channel : Subsystem
  FM_w : Outport  PortDimensions=6  VectorParamsAs1DForOutWhenUnconnected=off
  wires:
  Get Forces and Moments/1(FM_w) -> FM_w/1
  Bus Creator1/1 -> Get Forces and Moments/2(AeroCoeffs)
  Bus Selector7/2 -> Longitudinal Channel/2(Airpseed)  "<airspeed>"
  Bus Selector7/1 -> Longitudinal Channel/1(alpha)  "<alpha>"
  Bus Selector6/2 -> Lateral Channel/2(Airspeed)  "<airspeed>"
  Bus Selector6/1 -> Lateral Channel/1(beta)  "<beta>"
  Airdata/1 -> Bus Selector6/1, Bus Selector7/1, Get Forces and Moments/1(Airdata)
  Bus Selector2/1 -> Longitudinal Channel/3(dE)  "<dE>"
  Bus Selector1/2 -> Lateral Channel/4(dR)  "<dR>"
  Bus Selector1/1 -> Lateral Channel/3(dA)  "<dA>"
  CtrlSurfaces/1 -> Bus Selector1/1, Bus Selector2/1
  p,q,r/1 -> Lateral Channel/5(p,q,r), Longitudinal Channel/4(p,q,r)
  Lateral Channel/1(Lateral) -> Bus Creator1/1
  Longitudinal Channel/1(Longitudinal) -> Bus Creator1/2
  Bus Selector2/2 -> Longitudinal Channel/5(dA)  "<dA>"
  Bus Selector2/3 -> Longitudinal Channel/6(dR)  "<dR>"

== system eVTOL_System/Flight Controller/Autopilot/Fixed Wing Controller/Fixed Wing Controller Simulation/AER from Path Manager ==
  In1 : Inport
  Enable : EnablePort
  Out1 : Outport
  wires:
  In1/1 -> Out1/1

== system eVTOL_System/Flight Controller/Autopilot/Fixed Wing Controller/Fixed Wing Controller Simulation/Airspeed-Altitude Controller ==
  note: Airspeed and altitude are controlled independently
      | by ignoring their coupled dynamics.
  Airspeed SP : Inport
  Altitude SP : Inport  Port=2
  Climb Rate SP : Inport  Port=3
  Airspeed : Inport  Port=4
  xyz : Inport  Port=5
  vxyz : Inport  Port=6
  Enable : EnablePort  ShowOutputPort=on
  Airspeed Controller : slpidlib/PID Controller  Controller=PID  Form=Parallel  TimeDomain=Discrete-time  UseExternalTs=off  SampleTime=ControlSampleTime  IntegratorMethod=Trapezoidal  FilterMethod=Forward Euler  ControllerParametersSource=internal  P=FWControlParams.P_AIRSPD  I=FWControlParams.I_AIRSPD  UseKiTs=off  D=FWControlParams.D_AIRSPD  UseExternalDerivativeSource=off  N=FWControlParams.N_AIRSPD  UseFilter=on  TunerSelectOption=Transfer Function Based (PID Tuner App)  InitialConditionSource=internal  InitialConditionForIntegrator=0  InitialConditionForFilter=0  DifferentiatorICPrevScaledInput=0  ExternalReset=none  TrackingMode=off  Kt=1  LimitOutput=off  SatLimitsSource=internal  UpperSaturationLimit=Inf  LowerSaturationLimit=0  LinearizeAsGain=on  AntiWindupMode=clamping  Kb=1  LimitIntegrator=off  UpperIntegratorSaturationLimit=inf  LowerIntegratorSaturationLimit=-inf  POutMin=[]  POutMax=[]  IOutMin=[]  IOutMax=[]  DOutMin=[]  DOutMax=[]  NOutMin=[]  NOutMax=[]  SumOutMin=[]  SumOutMax=[]  SaturationOutMin=[]  SaturationOutMax=[]  PParamMin=[]  PParamMax=[]  IParamMin=[]  IParamMax=[]  DParamMin=[]  DParamMax=[]  NParamMin=[]  NParamMax=[]  KbParamMin=[]  KbParamMax=[]  KtParamMin=[]  KtParamMax=[]  KbOutMin=[]  KbOutMax=[]  KtOutMin=[]  KtOutMax=[]  IntegratorOutMin=[]  IntegratorOutMax=[]  FilterOutMin=[]  FilterOutMax=[]  SumI1OutMin=[]  SumI1OutMax=[]  SumI2OutMin=[]  SumI2OutMax=[]  SumI3OutMin=[]  SumI3OutMax=[]  SumI4OutMin=[]  SumI4OutMax=[]  SumDOutMin=[]  SumDOutMax=[]  DifferentiatorOutMin=[]  DifferentiatorOutMax=[]  FilterDiffOutCoefMin=[]  FilterDiffOutCoefMax=[]  ReciprocalOutMin=[]  ReciprocalOutMax=[]  SumDenOutMin=[]  SumDenOutMax=[]  SumNumOutMin=[]  SumNumOutMax=[]  DivideOutMin=[]  DivideOutMax=[]  UdiffTsProdOutMin=[]  UdiffTsProdOutMax=[]  NTsProdOutMin=[]  NTsProdOutMax=[]  UintegralTsProdOutMin=[]  UintegralTsProdOutMax=[]  UngainTsProdOutMin=[]  UngainTsProdOutMax=[]  ClampingZeroOutDataTypeStr=Inherit: Inherit via back propagation  ClampingZeroOutMin=[]  ClampingZeroOutMax=[]  FilterDenConstantOutDataTypeStr=Inherit: Inherit via back propagation  FilterDenConstantOutMin=[]  FilterDenConstantOutMax=[]  PCopyOutDataTypeStr=Inherit: Inherit via back propagation  PCopyOutMin=[]  PCopyOutMax=[]  NCopyOutDataTypeStr=Inherit: Inherit via back propagation  NCopyOutMin=[]  NCopyOutMax=[]  IntegratorContinuousStateAttributes=''  IntegratorStateMustResolveToSignalObject=off  IntegratorRTWStateStorageClass=Auto  FilterContinuousStateAttributes=''  FilterStateMustResolveToSignalObject=off  FilterRTWStateStorageClass=Auto  ParallelPVariant=InternalParameters  IdealPVariant=Disabled  IVariant=InternalParameters  DVariant=InternalParameters  IntegratorVariant=Discrete  SatVariant=Disabled  AWVariant=Passthrough  PCopyVariant=Disabled  TRVariant=Disabled  FdbkBlocksVariant=Forward  IdealPFdbkVariant=Disabled  SatFdbkVariant=Disabled  DerivativeFilterVariant=ForwardEulerFilter  NVariant=InternalParameters  NCopyVariant=Disabled  FilterICVariant=InternalICsFilter  IntegratorICVariant=InternalICs  ExternalResetVariant=Disabled  TRSumVariant=Passthrough  SumFdbkVariant=Disabled  SumVariant=Sum_PID  TsampFilterVariant=InternalTs  TsampNgainVariant=Passthrough  TsampIntegralVariant=Disabled_SignalSpec  ExternalSaturationOutDataTypeStr=Inherit: Same as second input  DerivativeSourceVariant=ErrorSignal  PreIntVariant=InternalPreInt
  Altitude controller : Subsystem
  Climb Rate SP Merge : Merge
  Climb Rate SP from Guidance : Subsystem  TreatAsAtomicUnit=on
  Compare To Constant : simulink/Logic and Bit Operations/Compare To Constant  relop===  const=uint8(1)  OutDataTypeStr=boolean
  Compare To Constant1 : simulink/Logic and Bit Operations/Compare To Constant  relop===  const=uint8(2)  OutDataTypeStr=boolean
  Pitch SP Controller : Subsystem
  Sum1 : Sum  Inputs=|+-
  Pitch SP : Outport
  Throttle : Outport  Port=2
  wires:
  Airspeed SP/1 -> Sum1/1
  Sum1/1 -> Airspeed Controller/1
  Airspeed/1 -> Sum1/2
  Airspeed Controller/1 -> Throttle/1
  Altitude SP/1 -> Altitude controller/1(Alt SP)
  xyz/1 -> Altitude controller/2(xyz)
  vxyz/1 -> Pitch SP Controller/2(vxyz)
  Pitch SP Controller/1(Pitch SP) -> Pitch SP/1
  Enable/1 -> Compare To Constant1/1, Compare To Constant/1
  Compare To Constant/1 -> Altitude controller/Enable
  Compare To Constant1/1 -> Climb Rate SP from Guidance/Enable
  Altitude controller/1(Climb Rate SP) -> Climb Rate SP Merge/1
  Climb Rate SP from Guidance/1(Out1) -> Climb Rate SP Merge/2
  Climb Rate SP Merge/1 -> Pitch SP Controller/1(Climb Rate SP)
  Climb Rate SP/1 -> Climb Rate SP from Guidance/1(Climb Rate SP)

== system eVTOL_System/Flight Controller/Autopilot/Fixed Wing Controller/Fixed Wing Controller Simulation/Attitude Controller ==
  YPR SP : Inport
  ypr : Inport  Port=2
  Ang Rate : Inport  Port=3
  Airspeed : Inport  Port=4
  Enable : EnablePort  ShowOutputPort=on
  AER Merge : Merge
  Compare To Constant : simulink/Logic and Bit Operations/Compare To Constant  relop===  const=uint8(1)  OutDataTypeStr=boolean
  Compare To Constant1 : simulink/Logic and Bit Operations/Compare To Constant  relop===  const=uint8(2)  OutDataTypeStr=boolean
  Demux1 : Demux  Outputs=3
  Pitch Roll Controller : Subsystem
  Rudder Heading Controller : Subsystem
  AER : Outport
  wires:
  ypr/1 -> Rudder Heading Controller/2(YPR), Pitch Roll Controller/3(YPR)
  YPR SP/1 -> Demux1/1
  Enable/1 -> Compare To Constant1/1, Compare To Constant/1
  AER Merge/1 -> AER/1
  Compare To Constant/1 -> Pitch Roll Controller/Enable
  Pitch Roll Controller/1(AER) -> AER Merge/1
  Rudder Heading Controller/1(AER) -> AER Merge/2
  Demux1/1 -> Rudder Heading Controller/1(Yaw SP)
  Demux1/2 -> Pitch Roll Controller/1(Pitch SP)
  Demux1/3 -> Pitch Roll Controller/2(Roll SP)
  Ang Rate/1 -> Rudder Heading Controller/3(Ang Rate), Pitch Roll Controller/4(Ang Rate)
  Compare To Constant1/1 -> Rudder Heading Controller/Enable
  Airspeed/1 -> Pitch Roll Controller/5(Airspeed)
